simulink model "s_dbpen_lqr"  (Simulink 7.8)
settings: Solver=ode1  StartTime=0.0  StopTime=inf  FixedStep=0.001  RelTol=1e-3
values from neighbouring files (symbols this model uses):
  A = [0 0 0 1 0 0 ... (first row only)    [DBPEN_ABCD_eqns.m]
  B = eta_g*Kg*eta_m*Kt/r_mp/Rm*B    [DBPEN_ABCD_eqns.m]
  C = eye(3,6)    [DBPEN_ABCD_eqns.m]    (also in setup_ip02_dbpen.m = eye(3,7))
  D = zeros(3,1)    [DBPEN_ABCD_eqns.m]
  K = [ 0 0 0 0 0 0 0 ]    [setup_ip02_dbpen.m]
  wcf_1 = 2 * pi * 50.0    (= 314.159265359)    [setup_ip02_dbpen.m]
  wcf_2 = 2 * pi * 10    (= 62.8318530718)    [setup_ip02_dbpen.m]
  X0 = [ 0 0.5*pi/180 0.5*pi/180 0 0 0 ]    [setup_ip02_dbpen.m]
  zetaf_1 = 0.9    [setup_ip02_dbpen.m]
  zetaf_2 = 0.9    [setup_ip02_dbpen.m]
undefined symbols (not defined in the file or in its folder): VMAX_AMP
libraries: simulink_extras x2
settings Model: Creator=Mfotoohi  LastModifiedBy=pmartin  SimulationMode=external  ExtModeTrigDuration=20000
settings SolverCC: PositivePriorityOrder=on
settings OptimizationCC: BooleanDataType=off  InitFltsAndDblsToZero=on
settings DebuggingCC: SaveWithParameterizedLinksMsg=none  FcnCallInpInsideContextMsg=Use local settings  StrictBusMsg=Warning
settings RTWCC: SystemTargetFile=quarc_windows.tlc  TemplateMakefile=quarc_default_tmf  Description=Quarc Win32 Target  ProcessScript=quarc_windows_make_rtw_hook
settings STFCustomTargetCC: TargetFcnLib=ansi_tfl_tmw.mat  TargetPreCompLibLocation=C:\PROGRA~2\QUARC\lib\2011b\windows\release  SystemTargetFile=quarc_windows.tlc
settings GRTTargetCC: TargetFcnLib=ansi_tfl_tmw.mat  TargetPreCompLibLocation=C:\PROGRA~2\QUARC\lib\2011b\windows\release  ParMdlRefBuildCompliant=off  CompOptLevelCompliant=off  ConcurrentExecutionCompliant=off  MatFileLogging=off  ExtMode=on  ExtModeMexFile=quarc_comm

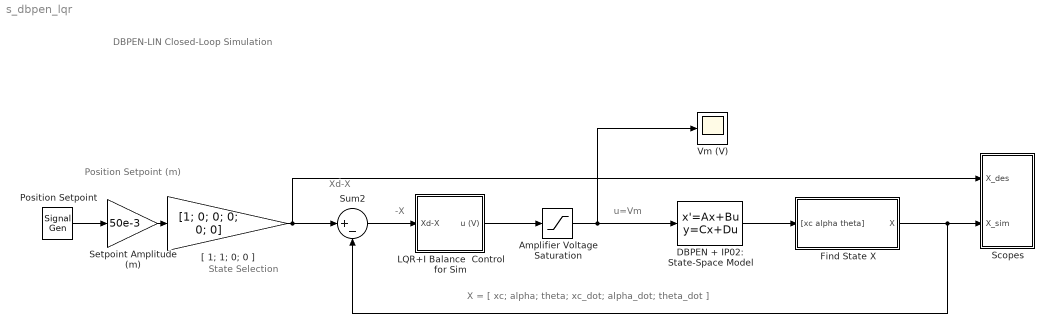
== system s_dbpen_lqr ==
  note: DBPEN-LIN Closed-Loop Simulation
  note: X = [ xc; alpha; theta; xc_dot; alpha_dot; theta_dot ]
  note: Xd-X
  note: State Selection
  note: Position Setpoint (m)
  note: u=Vm
  note: -X
  Amplifier Voltage Saturation : Saturate  UpperLimit=VMAX_AMP  LowerLimit=- VMAX_AMP
  DBPEN + IP02: State-Space Model : StateSpace  A=A  B=B  C=C  D=D  X0=[X0 0]
  Find State X : Subsystem
  LQR+I Balance  Control for Sim : Subsystem
  Position Setpoint : SignalGenerator  WaveForm=square  Frequency=0.05
  Scopes : Subsystem
  Setpoint Amplitude (m) : Gain  Gain=50e-3  SaturateOnIntegerOverflow=on  OutDataTypeStr=Inherit: Same as input  ParamDataTypeStr=Inherit: Same as input
  Sum2 : Sum  Inputs=|+-  SaturateOnIntegerOverflow=on  InputSameDT=on  OutDataTypeStr=Inherit: Same as first input
  Vm (V) : Scope
      settings: TimeRange=20  YMin=-10  YMax=10  SaveName=data_vm  DataFormat=Array  MaxDataPoints=20000
  "[ 1; 1; 0; 0 ]" : Gain  Gain=[1; 0; 0; 0; 0; 0]  SaturateOnIntegerOverflow=on  OutDataTypeStr=Inherit: Same as input  ParamDataTypeStr=Inherit: Same as input
  wires:
  "[ 1; 1; 0; 0 ]"/1 -> Scopes/1(X_des), Sum2/1
  Position Setpoint/1 -> Setpoint Amplitude (m)/1
  Setpoint Amplitude (m)/1 -> "[ 1; 1; 0; 0 ]"/1
  LQR+I Balance  Control for Sim/1(u (V)) -> Amplifier Voltage Saturation/1
  Sum2/1 -> LQR+I Balance  Control for Sim/1(Xd-X)
  Amplifier Voltage Saturation/1 -> DBPEN + IP02: State-Space Model/1, Vm (V)/1
  DBPEN + IP02: State-Space Model/1 -> Find State X/1("[xc alpha theta]")
  Find State X/1(X) -> Scopes/2(X_sim), Sum2/2

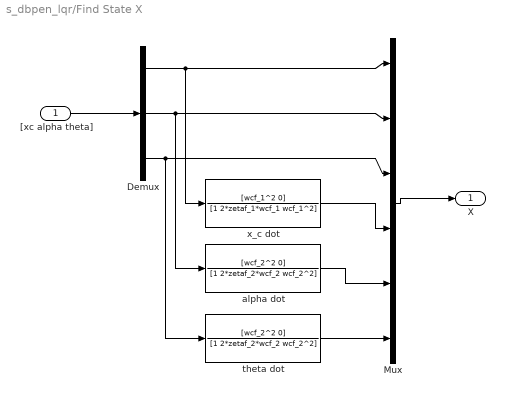
== system s_dbpen_lqr/Find State X ==
  "[xc alpha theta]" : Inport
  Demux : Demux  Outputs=3
  Mux : Mux  Inputs=6
  alpha dot : TransferFcn  Numerator=[wcf_2^2 0]  Denominator=[1 2*zetaf_2*wcf_2 wcf_2^2]
  theta dot : TransferFcn  Numerator=[wcf_2^2 0]  Denominator=[1 2*zetaf_2*wcf_2 wcf_2^2]
  x_c dot : TransferFcn  Numerator=[wcf_1^2 0]  Denominator=[1 2*zetaf_1*wcf_1 wcf_1^2]
  X : Outport
  wires:
  "[xc alpha theta]"/1 -> Demux/1
  Demux/1 -> Mux/1, x_c dot/1
  Demux/2 -> Mux/2, alpha dot/1
  Demux/3 -> Mux/3, theta dot/1
  x_c dot/1 -> Mux/4
  alpha dot/1 -> Mux/5
  theta dot/1 -> Mux/6
  Mux/1 -> X/1

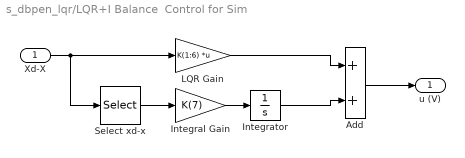
== system s_dbpen_lqr/LQR+I Balance  Control for Sim ==
  Xd-X : Inport
  Add : Sum
  Integral Gain : Gain  Gain=K(7)
  Integrator : Integrator  LimitOutput=on  UpperSaturationLimit=4  LowerSaturationLimit=-4
  LQR Gain : Gain  Gain=K(1:6)  Multiplication=Matrix(K*u)
  Select xd-x : Selector  InputPortWidth=6  IndexOptions=Index vector (dialog)  Indices=[1]  OutputSizes=1
  u (V) : Outport
  wires:
  Select xd-x/1 -> Integral Gain/1
  Add/1 -> u (V)/1
  Integrator/1 -> Add/2
  LQR Gain/1 -> Add/1
  Integral Gain/1 -> Integrator/1
  Xd-X/1 -> Select xd-x/1, LQR Gain/1

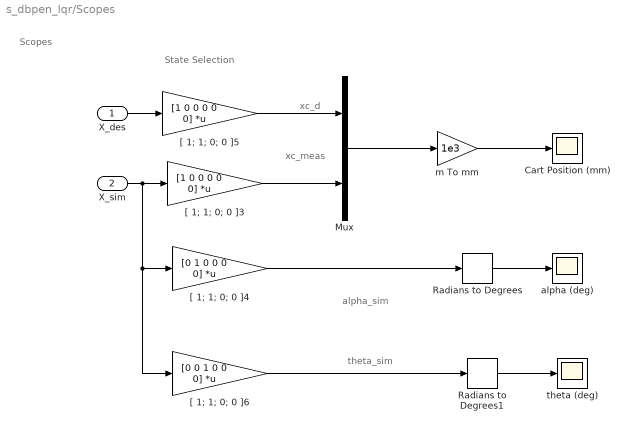
== system s_dbpen_lqr/Scopes ==
  note: xc_meas
  note: State Selection
  note: alpha_sim
  note: xc_d
  note: Scopes
  note: theta_sim
  X_des : Inport
  X_sim : Inport  Port=2
  Cart Position (mm) : Scope
      settings: TickLabels=on  TimeRange=20  YMin=-100  YMax=100  SaveName=data_xc  DataFormat=Array  MaxDataPoints=20000
  Mux : Mux  Inputs=2
  Radians to Degrees : simulink_extras/Transformations/Radians to Degrees
  Radians to Degrees1 : simulink_extras/Transformations/Radians to Degrees
  "[ 1; 1; 0; 0 ]3" : Gain  Gain=[1 0 0 0 0 0]  Multiplication=Matrix(K*u)  SaturateOnIntegerOverflow=on  OutDataTypeStr=Inherit: Same as input  ParamDataTypeStr=Inherit: Same as input
  "[ 1; 1; 0; 0 ]4" : Gain  Gain=[0 1 0 0 0 0]  Multiplication=Matrix(K*u)  SaturateOnIntegerOverflow=on  OutDataTypeStr=Inherit: Same as input  ParamDataTypeStr=Inherit: Same as input
  "[ 1; 1; 0; 0 ]5" : Gain  Gain=[1 0 0 0 0 0]  Multiplication=Matrix(K*u)  SaturateOnIntegerOverflow=on  OutDataTypeStr=Inherit: Same as input  ParamDataTypeStr=Inherit: Same as input
  "[ 1; 1; 0; 0 ]6" : Gain  Gain=[0 0 1 0 0 0]  Multiplication=Matrix(K*u)  SaturateOnIntegerOverflow=on  OutDataTypeStr=Inherit: Same as input  ParamDataTypeStr=Inherit: Same as input
  alpha (deg) : Scope
      settings: TickLabels=on  TimeRange=20  YMin=-10  YMax=10  SaveName=data_alpha  DataFormat=Array  MaxDataPoints=20000
  m To mm : Gain  Gain=1e3  SaturateOnIntegerOverflow=on  OutDataTypeStr=Inherit: Same as input  ParamDataTypeStr=Inherit: Same as input
  theta (deg) : Scope
      settings: TickLabels=on  TimeRange=20  YMin=-10  YMax=10  SaveName=data_theta  DataFormat=Array  MaxDataPoints=20000
  wires:
  Mux/1 -> m To mm/1
  m To mm/1 -> Cart Position (mm)/1
  X_des/1 -> "[ 1; 1; 0; 0 ]5"/1
  Radians to Degrees/1 -> alpha (deg)/1
  "[ 1; 1; 0; 0 ]5"/1 -> Mux/1
  "[ 1; 1; 0; 0 ]4"/1 -> Radians to Degrees/1
  Radians to Degrees1/1 -> theta (deg)/1
  "[ 1; 1; 0; 0 ]6"/1 -> Radians to Degrees1/1
  X_sim/1 -> "[ 1; 1; 0; 0 ]3"/1, "[ 1; 1; 0; 0 ]6"/1, "[ 1; 1; 0; 0 ]4"/1
  "[ 1; 1; 0; 0 ]3"/1 -> Mux/2
